simulink model "odesolve"  (R2020b)
settings: Solver=VariableStepAuto  StartTime=0.0  StopTime=10.0  RelTol=1e-3
settings Model: Creator=User  LastModifiedBy=User

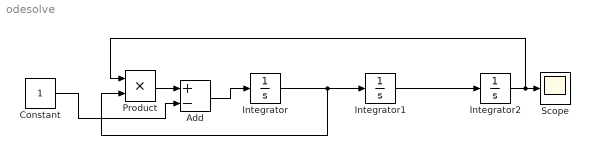
== system odesolve ==
  Add : Sum  Inputs=+-
  Constant : Constant
  Integrator : Integrator
  Integrator1 : Integrator
  Integrator2 : Integrator
  Product : Product
  Scope : Scope
  wires:
  Product/1 -> Add/1
  Integrator/1 -> Product/2, Integrator1/1
  Integrator2/1 -> Product/1, Scope/1
  Integrator1/1 -> Integrator2/1
  Add/1 -> Integrator/1
  Constant/1 -> Add/2
